simulink model "MotorControladoPorArmadura"  (R2016a)
settings: Solver=VariableStepAuto  StartTime=0.0  StopTime=10.0  RelTol=1e-3
values from neighbouring files (symbols this model uses):
  Bm = 0.050    (= 0.05)    [MotorControladoPorArmaduraVariables.m]
  Ea = 270    [MotorControladoPorArmaduraVariables.m]
  Jm = 0.4    [MotorControladoPorArmaduraVariables.m]
  KT = 1    [MotorControladoPorArmaduraVariables.m]
  La = 0.05    [MotorControladoPorArmaduraVariables.m]
  Ra = 1    [MotorControladoPorArmaduraVariables.m]
undefined symbols (not defined in the file or in its folder): Kb
settings Model: Creator=Abel  LastModifiedBy=Abel

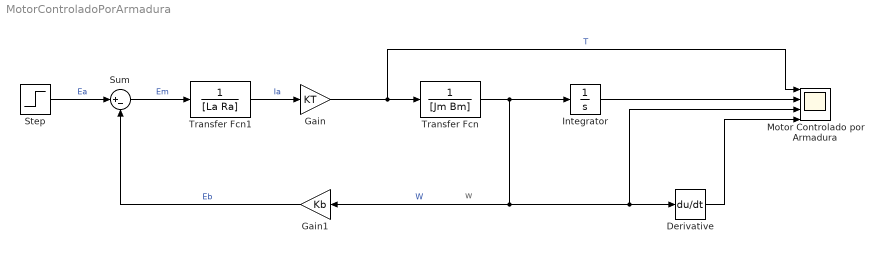
== system MotorControladoPorArmadura ==
  note: w
  Derivative : Derivative
  Gain : Gain  Gain=KT
  Gain1 : Gain  Gain=Kb
  Integrator : Integrator
  Motor Controlado por Armadura : Scope  NumInputPorts=4
  Step : Step  After=Ea  SampleTime=0
  Sum : Sum  Inputs=|+-
  Transfer Fcn : TransferFcn  Denominator=[Jm Bm]
  Transfer Fcn1 : TransferFcn  Denominator=[La Ra]
  wires:
  Gain/1 -> Motor Controlado por Armadura/1, Transfer Fcn/1  "T"
  Transfer Fcn1/1 -> Gain/1  "Ia"
  Transfer Fcn/1 -> Integrator/1, Derivative/1, Motor Controlado por Armadura/3, Gain1/1  "W"
  Sum/1 -> Transfer Fcn1/1  "Em"
  Gain1/1 -> Sum/2  "Eb"
  Step/1 -> Sum/1  "Ea"
  Integrator/1 -> Motor Controlado por Armadura/2
  Derivative/1 -> Motor Controlado por Armadura/4
